simulink model "predadorpresas"  (R2015a)
settings: Solver=ode45  StartTime=0.0  StopTime=simtime  FixedStep=step  RelTol=1e-3
values from neighbouring files (symbols this model uses):
  alfa1 = 1.4    [max_dif.m]    (also in primeirolab.m)
  alfa2 = V(1)    [max_dif.m]    (also in primeirolab.m = x(1))
  delta1 = 3.1    [max_dif.m]    (also in primeirolab.m)
  delta2 = -1.5    [max_dif.m]    (also in primeirolab.m)
  N1_0 = 4    [max_dif.m]    (also in primeirolab.m)
  N2_0 = V(2)    [max_dif.m]    (also in primeirolab.m = x(2))
settings Model: Creator=abran  LastModifiedBy=abran

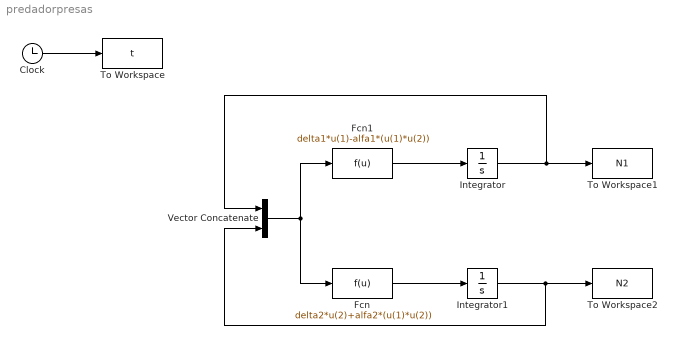
== system predadorpresas ==
  Clock : Clock
  Fcn : Fcn  Expr=delta2*u(2)+alfa2*(u(1)*u(2))
  Fcn1 : Fcn  Expr=delta1*u(1)-alfa1*(u(1)*u(2))
  Integrator : Integrator  InitialCondition=N1_0
  Integrator1 : Integrator  InitialCondition=N2_0
  To Workspace : ToWorkspace  VariableName=t  SampleTime=-1
  To Workspace1 : ToWorkspace  VariableName=N1  SampleTime=-1
  To Workspace2 : ToWorkspace  VariableName=N2  SampleTime=-1
  Vector Concatenate : Concatenate
  wires:
  Clock/1 -> To Workspace/1
  Fcn1/1 -> Integrator/1
  Fcn/1 -> Integrator1/1
  Integrator1/1 -> Vector Concatenate/2, To Workspace2/1
  Integrator/1 -> Vector Concatenate/1, To Workspace1/1
  Vector Concatenate/1 -> Fcn1/1, Fcn/1
